simulink model "ParrotRolling"  (R2020a)
settings: Solver=VariableStepAuto  StartTime=0.0  StopTime=10.0  RelTol=1e-3
settings Model: Creator=Fatih  LastModifiedBy=Fatih

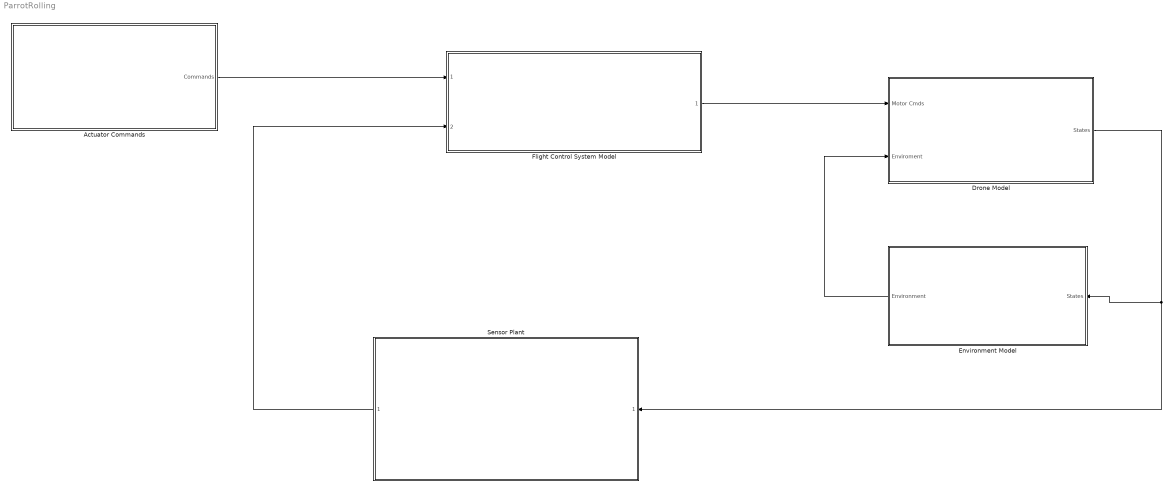
== system ParrotRolling ==
  Actuator Commands : Subsystem  Variant=on  VariantControlMode=Label  VariantControl=Choice  LabelModeActiveChoice=Choice
  Drone Model : Subsystem  Variant=on  VariantControl=Choice
  Environment Model : Subsystem  Variant=on  VariantControl=Choice
  Flight Control System Model : Subsystem  ReferencedSubsystem=FCS
  Sensor Plant : Subsystem  ReferencedSubsystem=Sensors
  wires:
  Flight Control System Model/1 -> Drone Model/1(Motor Cmds)
  Environment Model/1(Environment) -> Drone Model/2(Enviroment)
  Actuator Commands/1(Commands) -> Flight Control System Model/1
  Drone Model/1(States) -> Sensor Plant/1, Environment Model/1(States)
  Sensor Plant/1 -> Flight Control System Model/2

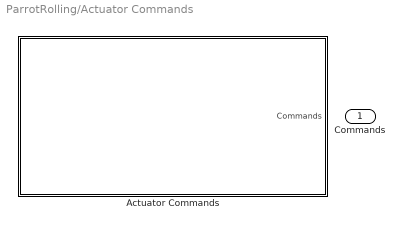
== system ParrotRolling/Actuator Commands ==
  Actuator Commands : Subsystem  VariantControl=Choice
  Commands : Outport

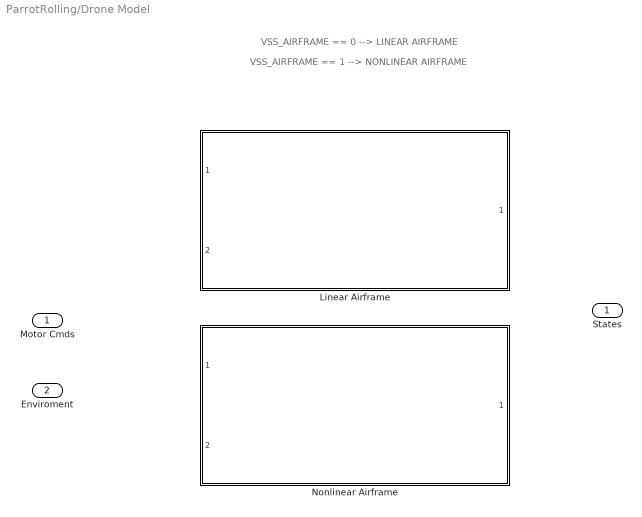
== system ParrotRolling/Drone Model ==
  note: VSS_AIRFRAME == 0 --> LINEAR AIRFRAME
  note: VSS_AIRFRAME == 1 --> NONLINEAR AIRFRAME
  Motor Cmds : Inport
  Enviroment : Inport  Port=2
  Linear Airframe : Subsystem  VariantControl="VSS_AIRFRAME  == 0"  ReferencedSubsystem=LinearAirframe
  Nonlinear Airframe : Subsystem  VariantControl=VSS_AIRFRAME == 1  ReferencedSubsystem=NonLinearAirframe
  States : Outport

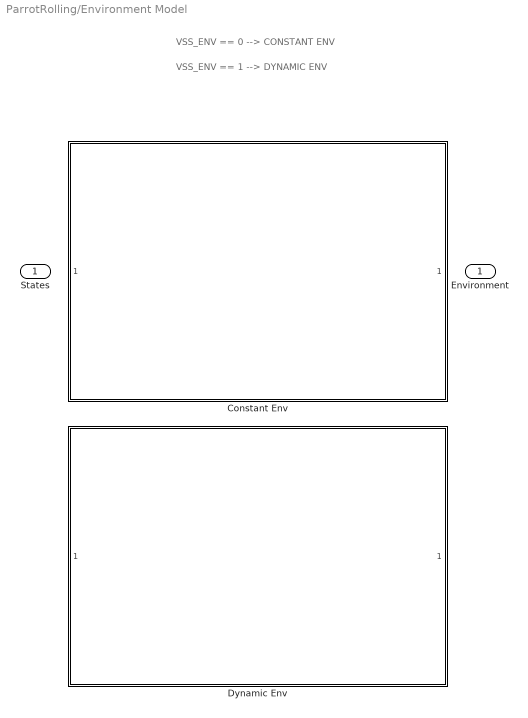
== system ParrotRolling/Environment Model ==
  note: VSS_ENV == 0 --> CONSTANT ENV
  note: VSS_ENV == 1 --> DYNAMIC ENV
  States : Inport
  Constant Env : Subsystem  VariantControl=VSS_ENV == 0  ReferencedSubsystem=ConstantEnvironment
  Dynamic Env : Subsystem  VariantControl=VSS_ENV == 1  ReferencedSubsystem=DynamicEnvironment
  Environment : Outport

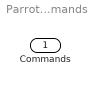
== system ParrotRolling/Actuator Commands/Actuator Commands ==
  Commands : Outport
